simulink model "a4_3_1_initial_function"  (R2018a)
settings: Solver=VariableStepAuto  StartTime=0.0  StopTime=10.0  RelTol=1e-3
InitFcn:
  | p = 10.78356;
Description:
  | An example of description
settings Model: Creator=r0x6f736f646f  LastModifiedBy=r0x6f736f646f

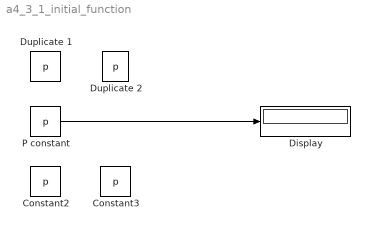
== system a4_3_1_initial_function ==
  Constant2 : Constant  Description=This block is a constant block  Value=p
  Constant3 : Constant  Description=This block is a constant block  Value=p
  Display : Display
  "Duplicate 1 " : Constant  Description=This block is a constant block  Value=p
  "Duplicate 2 " : Constant  Description=This block is a constant block  Value=p
  P constant : Constant  Description=This block is a constant block  Value=p
  wires:
  P constant/1 -> Display/1
